simulink model "JT9D_SS_Cantera_Template_org"  (Simulink 10.0)
settings: Solver=FixedStepDiscrete  StartTime=0.0  StopTime=1.5  FixedStep=0.015  RelTol=1e-3  EnableMultiTasking=on
libraries: Lib_TurboC_Duct_TMATSC x6, Lib_TurboC_Compressor_TMATSC x3, Lib_TurboC_Nozzle_TMATSC x2, Lib_Turbo_Shaft_TMATS x2, Lib_TurboC_Turbine_TMATSC x2, Lib_TurboC_Burner_TMATSC x1, Lib_TurboC_Ambient_TMATSC x1, Lib_TurboC_Inlet_TMATSC x1, Lib_TurboC_Splitter_TMATSC x1, Lib_Turbo_SFCCalc_TMATS x1, Lib_Solve_SSNRSolverJC_TMATS x1
CloseFcn:
  | run(strcat(MWS.top_level, filesep,'JT9D_SS_Cantera_Example_cleanup'))
settings Model: Creator=tlavelle  LastModifiedBy=bhisma
settings DataIOCC: LimitDataPoints=on
settings OptimizationCC: ExpressionDepthLimit=2147483647
settings DebuggingCC: SolverPrmCheckMsg=warning  StateNameClashWarn=warning
settings GRTTargetCC: GeneratePreprocessorConditionals=Disable all  CombineOutputUpdateFcns=on  GRTInterface=off
settings ConfigComp: CovExternalEMLEnable=off

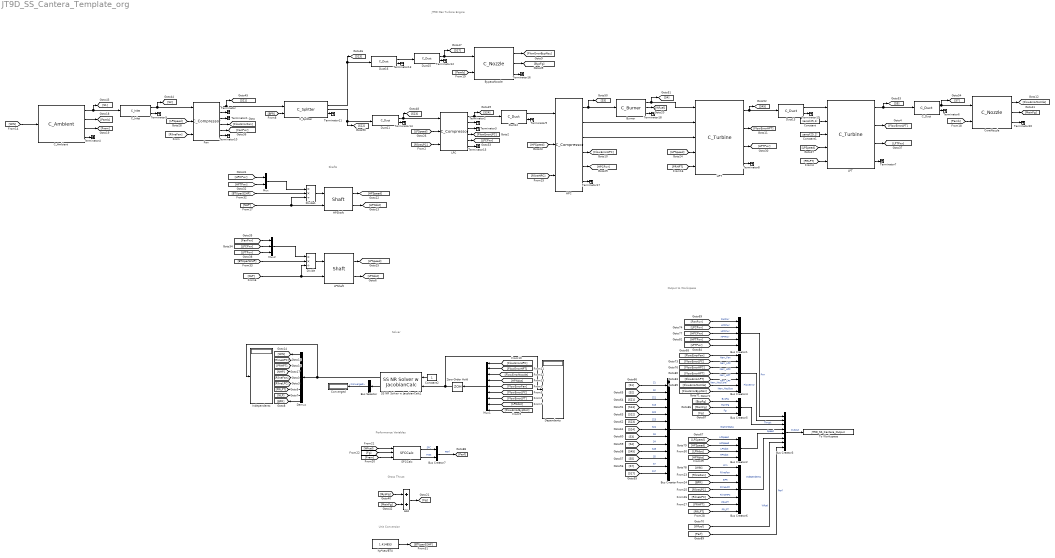
== system JT9D_SS_Cantera_Template_org ==
  note: Gross Thrust
  note: Performance Variables
  note: Solver
  note: Shafts
  note: Output to Workspace
  note: JT9D Gas Turbine Engine
  note: Unit Conversion
  Add : Sum
  "Burner " : Lib_TurboC_Burner_TMATSC/C_Burner   FAR_M=0.0187  hFuel_M=-1200  dP_M=.055
  Bus Creator : BusCreator  Inputs=13
  Bus Creator1 : BusCreator  Inputs=5
  Bus Creator2 : BusCreator  Inputs=4
  Bus Creator3 : BusCreator  Inputs=8
  Bus Creator4 : BusCreator  Inputs=7
  Bus Creator5 : BusCreator  Inputs=3
  Bus Creator6 : BusCreator  Inputs=7
  Bus Creator7 : BusCreator  Inputs=2
  Bus Selector : BusSelector  OutputSignals=Converged
  BypassNozzle : Lib_TurboC_Nozzle_TMATSC/C_Nozzle  Ath_in_M=0  Cfg_M=.9978  IDes_M=0  Wdes_M=562.61
  C_Ambient : Lib_TurboC_Ambient_TMATSC/C_Ambient  alt_M=100000  MN_M=0.85  dTs_M=0
  C_Duct : Lib_TurboC_Duct_TMATSC/C_Duct  dP_M=.01
  C_Inlet : Lib_TurboC_Inlet_TMATSC/C_Inlet  recovery_M=.995
  C_Splitter : Lib_TurboC_Splitter_TMATSC/C_Splitter
  Constant : Constant  Value=zeros(25,1)
  Constant1 : Constant  Value=zeros(25,1)
  Constant2 : Constant
  Converged : Display
  CoreNozzle : Lib_TurboC_Nozzle_TMATSC/C_Nozzle  Ath_in_M=0  Cfg_M=.9978  IDes_M=0  Wdes_M=113.51
  Demux : Demux  Outputs=9
  Dependents : Display
  Divide : Product  Inputs=**/
  Divide1 : Product  Inputs=**/
  Duct11 : Lib_TurboC_Duct_TMATSC/C_Duct  dP_M=.0025
  Duct12 : Lib_TurboC_Duct_TMATSC/C_Duct  dP_M=.0025
  Duct13 : Lib_TurboC_Duct_TMATSC/C_Duct  dP_M=.005
  Duct15 : Lib_TurboC_Duct_TMATSC/C_Duct  dP_M=.0075
  Duct16 : Lib_TurboC_Duct_TMATSC/C_Duct  dP_M=.0025
  Fan : Lib_TurboC_Compressor_TMATSC/C_Compressor  MapFile_M='FAN.map'  s_C_Nc_in_M=0  s_Wc_in_M=0  s_PR_in_M=0  s_eff_in_M=0  Wfrac1_M=0  hfrac1_M=1  Pfrac1_M=1  Wfrac2_M=0  hfrac2_M=1  Pfrac2_M=1  IDes_M=0  NcDes_M=100  effDes_M=.867  PRdes_M=1.645  RlineDes_M=2.3706
  HPC : Lib_TurboC_Compressor_TMATSC/C_Compressor  MapFile_M='HPC.map'  s_C_Nc_in_M=0  s_Wc_in_M=0  s_PR_in_M=0  s_eff_in_M=0  Wfrac1_M=.055  hfrac1_M=1  Pfrac1_M=1  Wfrac2_M=.035  hfrac2_M=1  Pfrac2_M=1  IDes_M=0  NcDes_M=100  effDes_M=.865  PRdes_M=5.609  RlineDes_M=2.0424
  HPShaft : Lib_Turbo_Shaft_TMATS/Shaft  Shaft_Inertia_M=1000
  HPT : Lib_TurboC_Turbine_TMATSC/C_Turbine  MapFile_M='HPT1.map'  s_C_Nc_M=0  s_Wc_M=0  s_PR_M=0  s_eff_M=0  BSW1_M=1  BSW2_M=0  IDes_M=0  Ndes_M=7499  PRmapDes_M=4.9299  effDes_M=.913  NcDes_M=100
  Independents : Display
  LPC : Lib_TurboC_Compressor_TMATSC/C_Compressor  MapFile_M='LPC.map'  s_C_Nc_in_M=0  s_Wc_in_M=0  s_PR_in_M=0  s_eff_in_M=0  Wfrac1_M=0  hfrac1_M=1  Pfrac1_M=1  Wfrac2_M=0  hfrac2_M=1  Pfrac2_M=1  IDes_M=0  NcDes_M=100  effDes_M=.868  PRdes_M=2.488  RlineDes_M=1.7664
  LPShaft : Lib_Turbo_Shaft_TMATS/Shaft  Shaft_Inertia_M=1000
  LPT : Lib_TurboC_Turbine_TMATSC/C_Turbine  MapFile_M='LPT.map'  s_C_Nc_M=0  s_Wc_M=0  s_PR_M=0  s_eff_M=0  BSW1_M=1  BSW2_M=1  IDes_M=0  Ndes_M=3723  PRmapDes_M=6.4203  effDes_M=.93  NcDes_M=100
  Mux : Mux  Inputs=2
  Mux1 : Mux  Inputs=9
  Mux2 : Mux  Inputs=3
  SFCCalc : Lib_Turbo_SFCCalc_TMATS/SFCCalc
  SS NR Solver w JacobianCalc1 : Lib_Solve_SSNRSolverJC_TMATS/SS NR Solver w JacobianCalc  SJac_Per_M=[1 .01 .01 10 .01 .01 .01 10 .01]  SNR_IC_M=[6742 2 2 7500 2 2 2 4000 5]  SNR_DX_M=10  SJacobianAttempts_M=5  Cond_Limits_M=.1
  Terminator{,1..20} (21 alike) : Terminator
  To Workspace : ToWorkspace  VariableName=JT9D_SS_Cantera_Output  SaveFormat=Timeseries  SampleTime=-1
  Zero-Order Hold : ZeroOrderHold  SampleTime=0.015
  hp*sec/BTU : Constant  Value=1.414853
  wires:
  HPC/1 -> [S3], "Burner "/1
  Mux1/1 -> Zero-Order Hold/1
  SS NR Solver w JacobianCalc1/1 -> Independents/1, Demux/1
  HPShaft/1 -> [HPSpeed]
  C_Splitter/1 -> Duct16/1, [S13]
  C_Inlet/1 -> Fan/1, [S2]
  HPT/1 -> Duct13/1, [S45]
  LPT/1 -> [S5], C_Duct/1
  Mux/1 -> Divide1/1
  Mux2/1 -> Divide/1
  LPShaft/1 -> [LPSpeed]
  Fan/4 -> [FlowErrorFan]
  [RlineFan] -> Fan/3
  Demux/5 -> [RlineFan]
  [FlowErrorFan] -> Mux1/5
  [RlineLPC] -> LPC/3
  [FlowErrorLPC] -> Mux1/6
  Demux/6 -> [RlineLPC]
  LPT/2 -> [FlowErrorLPT]
  [PRLPT] -> LPT/5
  Demux/7 -> [PRLPT]
  [FlowErrorLPT] -> Mux1/7
  [NLP] -> Divide/3, LPShaft/2
  LPShaft/2 -> [LPNdot]
  [LPNdot] -> Mux1/8
  Demux/8 -> [NLP]
  Demux/9 -> [BPR]
  [FlowErrorBypNoz] -> Mux1/9
  C_Ambient/1 -> [S1], C_Inlet/1
  [FlowErrorHPC] -> Mux1/1
  HPC/4 -> [FlowErrorHPC]
  [FlowErrorHPT] -> Mux1/2
  HPT/2 -> [FlowErrorHPT]
  CoreNozzle/1 -> [FlowErrorNozzle]
  [FlowErrorNozzle] -> Mux1/3
  HPShaft/2 -> [HPNdot]
  [HPNdot] -> Mux1/4
  [WIN] -> C_Ambient/1
  Demux/1 -> [WIN]
  [RlineHPC] -> HPC/3
  Demux/2 -> [RlineHPC]
  [PRHPT] -> HPT/5
  Demux/3 -> [PRHPT]
  Demux/4 -> [NHP]
  [NHP] -> Divide1/3, HPShaft/2
  C_Ambient/2 -> [Pamb]
  [Pamb] -> CoreNozzle/2
  C_Ambient/3 -> [Fram]
  [BPR] -> C_Splitter/2
  "Burner "/2 -> [Wfuel]
  [MainFg] -> Add/2
  Add/1 -> [Fg]
  [Fram] -> SFCCalc/3
  [Wfuel] -> SFCCalc/1
  [Fg] -> SFCCalc/2
  Bus Creator7/1 -> [Perf]  "Perf"
  LPC/4 -> [FlowErrorLPC]
  HPC/3 -> HPT/3
  HPC/2 -> HPT/2
  Fan/1 -> C_Splitter/1, [S21]
  C_Splitter/2 -> Duct11/1, [S22]
  Duct11/1 -> LPC/1, [S23]
  LPC/1 -> Duct12/1, [S24]
  Duct12/1 -> HPC/1
  Duct13/1 -> LPT/1
  C_Duct/1 -> CoreNozzle/1, [S7]
  Duct16/1 -> Duct15/1
  Duct15/1 -> BypassNozzle/1, [S17]
  [Pamb] -> BypassNozzle/2
  BypassNozzle/1 -> [FlowErrorBypNoz]
  [BypFg] -> Add/1
  Fan/2 -> Terminator/1
  Fan/3 -> Terminator1/1
  [HPSpeed] -> HPC/2
  [HPSpeed] -> HPT/4
  [LPSpeed] -> LPC/2
  [LPSpeed] -> LPT/4
  [LPSpeed] -> Fan/2
  LPC/2 -> Terminator2/1
  LPC/3 -> Terminator3/1
  HPT/3 -> [HPTPwr]
  HPC/5 -> [HPCPwr]
  [HPTPwr] -> Mux/2
  [HPCPwr] -> Mux/1
  LPC/5 -> [LPCPwr]
  [LPCPwr] -> Mux2/2
  [FanPwr] -> Mux2/1
  Fan/5 -> [FanPwr]
  LPT/3 -> [LPTPwr]
  [LPTPwr] -> Mux2/3
  BypassNozzle/2 -> [BypFg]
  CoreNozzle/2 -> [MainFg]
  Constant/1 -> LPT/2
  Constant1/1 -> LPT/3
  Zero-Order Hold/1 -> SS NR Solver w JacobianCalc1/2, Dependents/1
  C_Ambient/4 -> Terminator4/1
  C_Inlet/2 -> Terminator5/1
  "Burner "/1 -> [S4], HPT/1
  [S23] -> Bus Creator/6  "S23"
  [S22] -> Bus Creator/5  "S22"
  [S24] -> Bus Creator/7  "S24"
  [S3] -> Bus Creator/8  "S3"
  [S13] -> Bus Creator/4  "S13"
  [S4] -> Bus Creator/9  "S4"
  [S21] -> Bus Creator/3  "S21"
  [S45] -> Bus Creator/10  "S45"
  [S2] -> Bus Creator/2  "S2"
  [S1] -> Bus Creator/1  "S1"
  [S5] -> Bus Creator/11  "S5"
  [S7] -> Bus Creator/12  "S7"
  [S17] -> Bus Creator/13  "S17"
  Bus Creator/1 -> Bus Creator3/4  "StationData"
  Bus Creator2/1 -> Bus Creator3/5  "Speed"
  Bus Creator1/1 -> Bus Creator3/1  "Pwr"
  Bus Creator3/1 -> To Workspace/1  "Output"
  SFCCalc/1 -> Bus Creator7/1  "SFC"
  SFCCalc/2 -> Bus Creator7/2  "Fnet"
  CoreNozzle/3 -> Terminator20/1
  HPC/6 -> Terminator17/1
  Fan/6 -> Terminator10/1
  C_Splitter/3 -> Terminator11/1
  Duct15/2 -> Terminator12/1
  Duct16/2 -> Terminator13/1
  Duct11/2 -> Terminator14/1
  LPC/6 -> Terminator15/1
  BypassNozzle/3 -> Terminator16/1
  Duct12/2 -> Terminator9/1
  HPT/4 -> Terminator8/1
  "Burner "/3 -> Terminator18/1
  LPT/4 -> Terminator7/1
  Duct13/2 -> Terminator19/1
  C_Duct/2 -> Terminator6/1
  Bus Selector/1 -> Converged/1  "<Converged>"
  SS NR Solver w JacobianCalc1/2 -> Bus Selector/1
  [FlowErrorFan] -> Bus Creator4/1  "Nerr_Fan"
  [FlowErrorBypNoz] -> Bus Creator4/7  "Nerr_NozByp"
  [FlowErrorLPC] -> Bus Creator4/2  "Nerr_LPC"
  [FlowErrorHPC] -> Bus Creator4/3  "Nerr_HPC"
  [FlowErrorHPT] -> Bus Creator4/4  "Nerr_HPT"
  [FlowErrorLPT] -> Bus Creator4/5  "Nerr_LPT"
  [FlowErrorNozzle] -> Bus Creator4/6  "Nerr_NozCore"
  [FanPwr] -> Bus Creator1/1  "FanPwr"
  [LPCPwr] -> Bus Creator1/2  "LPCPwr"
  [HPCPwr] -> Bus Creator1/3  "HPCPwr"
  [HPTPwr] -> Bus Creator1/4  "HPTPwr"
  [LPTPwr] -> Bus Creator1/5
  [BypFg] -> Bus Creator5/1  "BypFg"
  [MainFg] -> Bus Creator5/2  "MainFg"
  [Fg] -> Bus Creator5/3  "Fg"
  [Perf] -> Bus Creator3/8  "Perf"
  [LPSpeed] -> Bus Creator2/1  "LPSpeed"
  [HPSpeed] -> Bus Creator2/2  "HPSpeed"
  [LPNdot] -> Bus Creator2/3  "LPNdot"
  [HPNdot] -> Bus Creator2/4  "HPNdot"
  [PRHPT] -> Bus Creator6/6  "PRHPT"
  [RlineHPC] -> Bus Creator6/5  "RlineHPC"
  [RlineFan] -> Bus Creator6/2  "RlineFan"
  [BPR] -> Bus Creator6/3  "BPR"
  [RlineLPC] -> Bus Creator6/4  "RlineLPC"
  [PRLPT] -> Bus Creator6/7  "PRLPT"
  [WIN] -> Bus Creator6/1  "Win"
  Bus Creator4/1 -> Bus Creator3/2  "FlowError"
  Bus Creator5/1 -> Bus Creator3/3  "Thrust"
  Bus Creator6/1 -> Bus Creator3/6  "Independents"
  [Wfuel] -> Bus Creator3/7  "Wfuel"
  Divide/1 -> LPShaft/1
  Divide1/1 -> HPShaft/1
  [BTUperS2HP] -> Divide1/2
  [BTUperS2HP] -> Divide/2
  hp*sec/BTU/1 -> [BTUperS2HP]
  Constant2/1 -> SS NR Solver w JacobianCalc1/1
